simulink model "Priview_PID"  (Simulink 8.4)
settings: Solver=ode45  StartTime=0.0  StopTime=80  FixedStep=0.1  RelTol=1e-3
libraries: Solver_SF x1
settings Model: Creator=强哥  LastModifiedBy=强哥
settings DataIOCC: SignalLoggingSaveFormat=Dataset
settings OptimizationCC: ExpressionDepthLimit=128
settings DebuggingCC: UnderspecifiedInitializationDetection=Simplified  MergeDetectMultiDrivingBlocksExec=error  FcnCallInpInsideContextMsg=EnableAllAsError  StateNameClashWarn=none
settings GRTTargetCC: CombineOutputUpdateFcns=on  GRTInterface=off

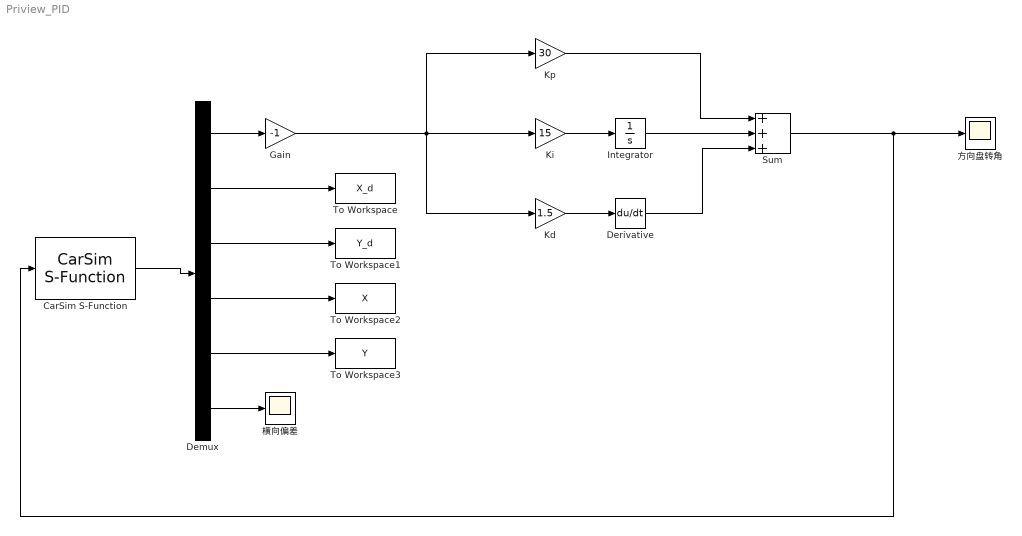
== system Priview_PID ==
  CarSim S-Function : Solver_SF/CarSim S-Function  Priority=1  VehicleCode=i_i  SIMFILE=simfile
  Demux : Demux  Outputs=6
  Derivative : Derivative
  Gain : Gain  Gain=-1
  Integrator : Integrator
  Kd : Gain  Gain=1.5
  Ki : Gain  Gain=15
  Kp : Gain  Gain=30
  Sum : Sum  Inputs=+++
  To Workspace : ToWorkspace  VariableName=X_d  SampleTime=-1
  To Workspace1 : ToWorkspace  VariableName=Y_d  SampleTime=-1
  To Workspace2 : ToWorkspace  VariableName=X  SampleTime=-1
  To Workspace3 : ToWorkspace  VariableName=Y  SampleTime=-1
  方向盘转角 : Scope
      settings: YMin=0  YMax=100
  横向偏差 : Scope
      settings: YMin=-0.6  YMax=0.6
  wires:
  CarSim S-Function/1 -> Demux/1
  Demux/6 -> 横向偏差/1
  Demux/1 -> Gain/1
  Demux/2 -> To Workspace/1
  Demux/3 -> To Workspace1/1
  Demux/4 -> To Workspace2/1
  Demux/5 -> To Workspace3/1
  Ki/1 -> Integrator/1
  Kd/1 -> Derivative/1
  Gain/1 -> Kd/1, Kp/1, Ki/1
  Integrator/1 -> Sum/2
  Kp/1 -> Sum/1
  Derivative/1 -> Sum/3
  Sum/1 -> CarSim S-Function/1, 方向盘转角/1
